simulink model "lineChanging_backup"  (R2016b)
settings: Solver=VariableStepAuto  StartTime=0  StopTime=5  MaxStep=0.05  RelTol=1e-3
model workspace (MAT data in the model file):
  FARAWAY = Simulink.Parameter
  FARAWAY.Value = 100
  FARAWAY.DataType = 'auto'
  FARAWAY.Dimensions = [1 1]
  MIN_SAFE_DIST = Simulink.Parameter
  MIN_SAFE_DIST.Value = 1
  MIN_SAFE_DIST.DataType = 'auto'
  MIN_SAFE_DIST.Dimensions = [1 1]
  WORLD_SIZE = Simulink.Parameter
  WORLD_SIZE.Value = 12
  WORLD_SIZE.DataType = 'auto'
  WORLD_SIZE.Dimensions = [1 1]
  dt = Simulink.Parameter
  dt.Value = 0.05
  dt.DataType = 'auto'
  dt.Dimensions = [1 1]
values from neighbouring files (symbols this model uses):
  WORLD_SIZE = 12    [stateflowSim.m]
settings Model: Creator=larry  LastModifiedBy=larry

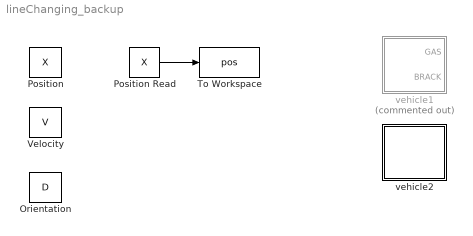
== system lineChanging_backup ==
  Orientation : DataStoreMemory  DataStoreName=D  WriteAfterReadMsg=warning  InitialValue=[1 1; 0 0]  ShowAdditionalParam=off  OutDataTypeStr=double
  Position : DataStoreMemory  DataStoreName=X  InitialValue=[-0.5 6; -0.5 1.5]  ShowAdditionalParam=off  OutDataTypeStr=double
  Position Read : DataStoreRead  DataStoreName=X
  To Workspace : ToWorkspace  VariableName=pos  SampleTime=-1
  Velocity : DataStoreMemory  DataStoreName=V  InitialValue=[1 1.5; 0 0]  ShowAdditionalParam=off  OutDataTypeStr=double
  vehicle1 : Stateflow chart  Commented=on  TreatAsAtomicUnit=on
  vehicle2 : Stateflow chart  TreatAsAtomicUnit=on
  wires:
  Position Read/1 -> To Workspace/1

== stateflow chart lineChanging_backup/vehicle2 ==
  state Straight
    en:
    safeDist = max(norm(V(:,this))*1,MIN_SAFE_DIST);
    du:
    safeDist = max(norm(V(:,this))*1,MIN_SAFE_DIST);
    state Follow
      en:
      [dxfr, dvfr] = frontCarInfo();
      du:
      [dxfr, dvfr] = frontCarInfo();
      state Safe
        du:
        if dvfr < 0
        accelerateDrive();
        else
        slowDownDrive();
        end
      state Dangerous
        du:
        slowDownDrive();
      Safe -> Dangerous : [dxfr < 1.6*safeDist]
      Dangerous -> Safe : [dxfr > 2*safeDist]
      (default) -> Dangerous [order 2]
      (default) -> Safe [order 1] : [dxfr > 2*safeDist]
    state FreeDriving
      state Accelerate
        du:
        accelerateDrive();
      state FixRate
        en:
        setRateTo(VEC_MAX);
        du:
        fixedRateDrive();
      (default) -> Accelerate [order 2]
      Accelerate -> FixRate : [reach(VEC_MAX)]
      (default) -> FixRate [order 1] : [reach(VEC_MAX)]
    (default) -> Follow [order 1] : [hasFrontCar()]
    (default) -> FreeDriving [order 2]
    FreeDriving -> Follow : [hasFrontCar()]
    Follow -> FreeDriving : [frontCarHasLeft()]
  data: res function_output; res function_output; res function_output; target function_input; target function_input; dx function_output; dv function_output; idx function_output; X data_store_memory; this local uint8 size=1 =uint8(2); ACC_MAX constant double =2.5; D data_store_memory; VEC_MAX constant double =2.5; V data_store_memory; MIN_SAFE_DIST parameter; WORLD_SIZE parameter; dt parameter; dxfr local; dvfr local; safeDist local; FARAWAY parameter
  function slowDownDrive:
    | function slowDownDrive
    |  
    | x = X(:,this);
    | v = V(:,this);
    | a = D(:,this) * (-ACC_MAX);
    | 
    | x = x + v * dt + 0.5 * a * dt * dt;
    | v = v + a * dt;
    | 
    | % a rounded world
    | if x(1) > WORLD_SIZE
    |     x(1) = -WORLD_SIZE;
    | elseif x(1) < -WORLD_SIZE
    |     x(1) = WORLD_SIZE;
    | elseif x(2) > WORLD_SIZE
    |     x(2) = -WORLD_SIZE;
    | elseif x(2) < -WORLD_SIZE
    |     x(2) = WORLD_SIZE;
    | end
    | 
    | X(:,this) = x;
    | V(:,this) = v;
  function res = hasFrontCar:
    | function res = hasFrontCar
    | 
    | % constants
    | THRES = 2.25 * safeDist;
    | RANGE = 2 * WORLD_SIZE;
    | 
    | res = false;
    | 
    | % row of X: coordinate, col of X: num of cars
    | num = size(X, 2);
    | if num == 1
    |     return;
    | end
    | 
    | dx = ones(num, 1)*FARAWAY;
    | x = X(:,this);
    | d = D(:,this);
    | carSize = [0.3; 0.4];
    | 
    | for k=1:length(dx)
    |     
    |     if k ~= this
    |         % compute difference
    |         xdelta = X(:,k) - x;
    |     
    |         % parallel and vertical distance
    |         delta_p = dot(xdelta, d);
    |         delta_v = norm(xdelta - (d * delta_p));
    |     
    |         % vertical distance is larger than car width
    |         if delta_v < carSize(1)
    |             dx(k) = delta_p;
    |       
    |             % a rounded world
    |             dx(k) = mod((dx(k)+RANGE), RANGE);
    |         end
    |     end
    | end
    | 
    | % set zero dX to a large enough value
    | closest = min(dx);
    | res = closest <= THRES;
  function res = frontCarHasLeft:
    | function res = frontCarHasLeft
    | 
    | % Constants 
    | THRES = 2.5 * safeDist;
    | RANGE = 2 * WORLD_SIZE;
    | 
    | % if only one car in the environment return directly
    | res = true;
    | num = size(X, 1);
    | if num == 1
    |     return;
    | end
    | 
    | % get the closet car index and its distance
    | dx = zeros(num, 1);
    | x = X(:,this);
    | d = D(:,this);
    | car_size = [0.3; 0.4];
    | 
    | for k=1:length(dx)
    |     
    |     xdelta = X(:,k) - x;
    |     xdelta_p = dot(xdelta, d);                  % parallel component
    |     xdelta_v = norm(xdelta - (d * xdelta_p));   % vertical component
    |     
    |     % when the vertical component is larger than the car width
    |     if xdelta_v < car_size(1)
    |         dx(k) = xdelta_p;
    |         % since we are in the round world, normalize the distance if the 
    |         % front car is behind us 
    |         % a rounded world
    |         dx(k) = mod((dx(k)+RANGE), RANGE);
    |     else
    |         dx(k) = FARAWAY;
    |     end
    | end
    | 
    | % set the zero dx to a large enough value for convenience
    | dx(dx == 0) = FARAWAY;
    | closest = min(dx);
    | res = closest > THRES;
  function res = reach(target):
    | function res = reach(target)
    | 
    | res = abs(target - norm(V(:,this))) < 0.125;
  function accelerateDrive:
    | function accelerateDrive
    | 
    | x = X(:,this);
    | v = V(:,this);
    | a = D(:,this) * ACC_MAX;
    | 
    | x = x + v * dt + 0.5 * a * dt * dt;
    | v = v + a * dt;
    | 
    | % a rounded world
    | if x(1) > WORLD_SIZE
    |     x(1) = -WORLD_SIZE;
    | elseif x(1) < -WORLD_SIZE
    |     x(1) = WORLD_SIZE;
    | elseif x(2) > WORLD_SIZE
    |     x(2) = -WORLD_SIZE;
    | elseif x(2) < -WORLD_SIZE
    |     x(2) = WORLD_SIZE;
    | end
    | 
    | X(:,this) = x;
    | V(:,this) = v;
  function fixedRateDrive:
    | function fixedRateDrive
    | 
    | x = X(:,this);
    | v = V(:,this);
    | 
    | % update new position
    | x = x + v * dt;
    | 
    | % a rounded world
    | if x(1) > WORLD_SIZE
    |     x(1) = -WORLD_SIZE;
    | elseif x(1) < -WORLD_SIZE
    |     x(1) = WORLD_SIZE;
    | elseif x(2) > WORLD_SIZE
    |     x(2) = -WORLD_SIZE;
    | elseif x(2) < -WORLD_SIZE
    |     x(2) = WORLD_SIZE;
    | end
    | 
    | X(:,this) = x;
  function setRateTo(target):
    | function setRateTo(target)
    | 
    | V(:,this) = D(:,this) * target;
  function [dx,dv] = frontCarInfo:
    | function [dx,dv] = frontCarInfo()
    | 
    | index = frontCarIndex();
    | 
    | x = X(:,this);
    | v = V(:,this);
    | d = D(:,this);
    | 
    | xfront = X(:,index);
    | vfront = V(:,index);
    | 
    | range = 2 * WORLD_SIZE;
    | 
    | dx = mod((dot(xfront - x, d)+range), range);
    | dv = dot(vfront-v, d);
    | 
    | end
  function idx = frontCarIndex:
    | function idx = frontCarIndex
    | 
    | RANGE = 2*WORLD_SIZE;
    | 
    | dx = ones(size(X, 2), 1)*FARAWAY;
    | x = X(:,this);
    | v = V(:,this);
    | d = D(:,this);
    | 
    | for k=1:length(dx)
    |     xk = X(:,k);
    |     if k ~= this && (abs(xk(2)-x(2)) < 1)
    |         dx(k) = dot(xk - x, d);
    |         dx(k) = mod((dx(k)+RANGE), RANGE);
    |     end
    | end
    | 
    | % set zero dx to a large enough value
    | [~, idx] = min(dx);
    | idx = uint8(idx);
    | 
    | end

== stateflow chart lineChanging_backup/vehicle1 ==
  state Start
    en:
    GAS.data = [0;2.5];
    BRACK.data = [0;2.5];
  state Straight
    state ClearFront
      en:
      GAS.data(1) = V_MAX;
      send(GAS);
    state HasFrontCar
    (default) -> ClearFront [order 2]
    (default) -> HasFrontCar [order 1] : [hasFrontCar()]
    HasFrontCar -> ClearFront : [frontCarHasLeft()]
    ClearFront -> HasFrontCar : [hasFrontCar()]
  (default) -> Start
  Start -> Straight
  data: res function_output; res function_output; idx function_output; this local uint8 size=1 =1; X data_store_memory; V data_store_memory; GAS output; BRACK output; V_MAX constant double =2.5; WORLD_SIZE parameter; MIN_SAFE_DIST parameter; FARAWAY parameter
  function res = hasFrontCar:
    | function res = hasFrontCar()
    | 
    | res = false;
    | 
    | % define constants here
    | THRES = 2.25 * MIN_SAFE_DIST;
    | RANGE = 2 * WORLD_SIZE;
    | 
    | % a column vector is a coordinate, the number of column is equals to
    | % the number of cars
    | num = size(X, 2);
    | if num == 1
    |     return;
    | end
    | 
    | % internal states
    | x = X(:,this);
    | d = D(:,this);
    | carSize = [0.3; 0.4];
    | 
    | distance = zeros(num, 1);
    | for k=1:length(distance)
    |     
    |     % compute difference
    |     xdelta = X(:,k) - x;
    |     
    |     % parallel and vertical distance
    |     delta_p = dot(xdelta, d);
    |     delta_v = norm(xdelta - (d * delta_p));
    |     
    |     % vertical distance is larger than car width
    |     if delta_v < carSize(1)
    |         distance(k) = delta_p;
    |     else
    |         distance(k) = FARAWAY;
    |     end
    |     
    |     % a rounded world
    |     distance(k) = mod((distance(k)+RANGE), RANGE);
    | end
    | 
    | % set zero dX to a large enough value
    | distance(distance == 0) = FARAWAY;
    | closest = min(distance);
    | res = closest <= THRES;
  function res = frontCarHasLeft:
    | function res = frontCarHasLeft()
    | 
    | % Constants 
    | THRES = 2.5 * MIN_SAFE_DIST;
    | RANGE = 2 * WORLD_SIZE;
    | 
    | % if only one car in the environment return directly
    | res = true;
    | num = size(X, 1);
    | if num == 1
    |     return;
    | end
    | 
    | % get the closet car index and its distance
    | dx = zeros(num, 1);
    | x = X(:,this);
    | d = D(:,this);
    | car_size = [0.3; 0.4];
    | 
    | for k=1:length(dx)
    |     
    |     xdelta = X(:,k) - x;
    |     xdelta_p = dot(xdelta, d);                  % parallel component
    |     xdelta_v = norm(xdelta - (d * xdelta_p));   % vertical component
    |     
    |     % when the vertical component is larger than the car width
    |     if xdelta_v < car_size(1)
    |         dx(k) = xdelta_p;
    |     else
    |         dx(k) = FARAWAY;
    |     end
    |     
    |     % since we are in the round world, normalize the distance if the 
    |     % front car is behind us 
    |     % a rounded world
    |     dx(k) = mod((dx(k)+RANGE), RANGE);
    | end
    | 
    | % set the zero dx to a large enough value for convenience
    | dx(dx == 0) = FARAWAY;
    | closest = min(dx);
    | res = closest > THRES;
  function idx = frontCarIndex:
    | function idx = frontCarIndex()
    | 
    | RANGE = 2*WORLD_SIZE;
    | 
    | dx = zeros(size(X, 2), 1);
    | x = X(:,this);
    | v = V(:,this);
    | d = D(:,this);
    | 
    | for k=1:length(dx)
    |     dx(k) = dot(X(:,k) - x, d);
    |     dx(k) = mod((dx(k)+RANGE), RANGE);
    | end
    | 
    | % set zero dX to a large enough value
    | dx(dx == 0) = FARAWAY;
    | [~, idx] = min(dx);
    | idx = uint8(idx);
